simulink model "SS"  (R2017a)
settings: Solver=VariableStepAuto  StartTime=0.0  StopTime=50  RelTol=1e-3
values from neighbouring files (symbols this model uses):
  Ad = sysdd.A    [trock.m]
  Bd = sysdd.B(1:2)    [trock.m]
  C11 = [ C1(2,:); C1(4,:)]    [trock.m]
  Cd = sysdd.C    [trock.m]
  Dd = sysdd.D(:,1:2)    [trock.m]
  Ed = sysdd.B(3:4)    [trock.m]
  Kd = sysdd.D(:,3:4)    [trock.m]
  M_c = B_1 * A * B_1'    [trock.m]
  N_c = [ N(:,5) N(:,6)]    [trock.m]
  Ts = 0.566    [trock.m]
undefined symbols (not defined in the file or in its folder): Ac, Bc, Cc, Dc, Ec, Kc
libraries: powerlib_meascontrol x2
settings Model: Creator=CBalla  LastModifiedBy=nvink

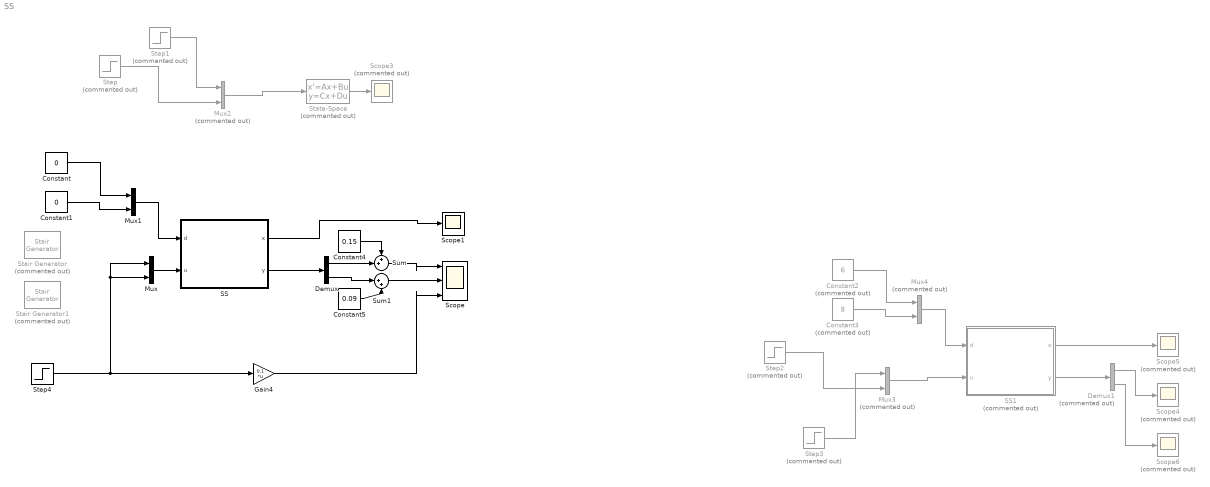
== system SS ==
  Constant : Constant  Value=0
  Constant1 : Constant  Value=0
  Constant2 : Constant  Commented=on  Value=6
  Constant3 : Constant  Commented=on  Value=8
  Constant4 : Constant  Value=0.15
  Constant5 : Constant  Value=0.09
  Demux : Demux  Outputs=2
  Demux1 : Demux  Commented=on  Outputs=2
  Gain4 : Gain  Gain=0.1  Multiplication=Matrix(K*u)
  Mux : Mux  Inputs=2
  Mux1 : Mux  Inputs=2
  Mux2 : Mux  Commented=on  Inputs=2
  Mux3 : Mux  Commented=on  Inputs=2
  Mux4 : Mux  Commented=on  Inputs=2
  SS : Subsystem
  SS1 : Subsystem  Commented=on
  Scope : Scope  NumInputPorts=3
  Scope1 : Scope
  Scope{3..6} (4 alike) : Scope  Commented=on
  Stair Generator : powerlib_meascontrol/Pulse & Signal Generators/Stair Generator  Commented=on  t=[0, 5, 10, 15, 20, 25, 30, 35, 40, 45]  e=[0, 1, 2, 3, 4 ,4 , 3, 2, 1,0]  Ts=0
      settings: SourceProductName=Simscape Power Systems
  Stair Generator1 : powerlib_meascontrol/Pulse & Signal Generators/Stair Generator  Commented=on  t=[0, 5, 10,15]  e=[0, 0.1, 0.2,0.4]  Ts=0
      settings: SourceProductName=Simscape Power Systems
  State-Space : StateSpace  Commented=on  A=-M_c  B=N_c  C=C11  D=[0, 0;0 ,0 ]  X0=0
  Step : Step  Commented=on  SampleTime=0
  Step1 : Step  Commented=on  Time=3  SampleTime=0
  Step2 : Step  Commented=on  SampleTime=0
  Step3 : Step  Commented=on  Time=15  SampleTime=0
  Step4 : Step  Time=5  After=0.4  SampleTime=0
  Sum : Sum  Inputs=++|
  Sum1 : Sum  Inputs=|++
  wires:
  SS/1(x) -> Scope1/1
  Mux/1 -> SS/2(u)
  Mux1/1 -> SS/1(d)
  Constant/1 -> Mux1/1
  Constant1/1 -> Mux1/2
  SS/2(y) -> Demux/1
  Mux2/1 -> State-Space/1
  State-Space/1 -> Scope3/1
  Step1/1 -> Mux2/1
  Step/1 -> Mux2/2
  SS1/1(x) -> Scope5/1
  Mux4/1 -> SS1/1(d)
  Constant2/1 -> Mux4/1
  Constant3/1 -> Mux4/2
  SS1/2(y) -> Demux1/1
  Demux1/1 -> Scope4/1
  Demux1/2 -> Scope6/1
  Mux3/1 -> SS1/2(u)
  Step3/1 -> Mux3/1
  Step2/1 -> Mux3/2
  Demux/1 -> Sum/2
  Demux/2 -> Sum1/1
  Constant4/1 -> Sum/1
  Constant5/1 -> Sum1/2
  Sum/1 -> Scope/1
  Sum1/1 -> Scope/2
  Step4/1 -> Gain4/1, Mux/1, Mux/2
  Gain4/1 -> Scope/3

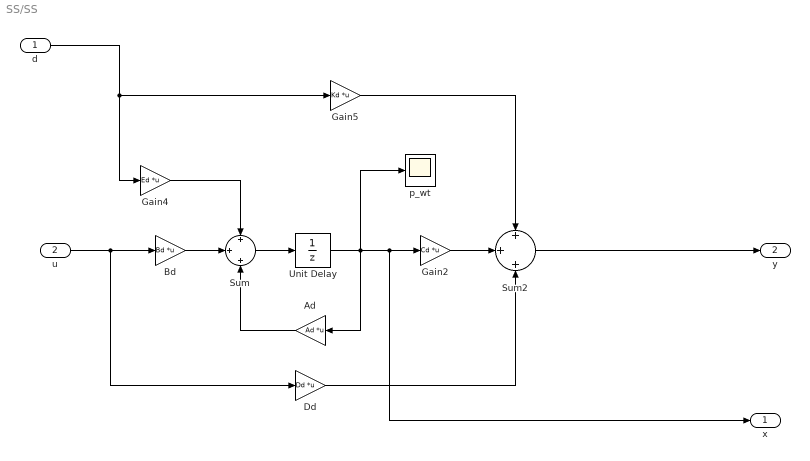
== system SS/SS ==
  d : Inport
  u : Inport  Port=2
  Ad : Gain  Gain=Ad  Multiplication=Matrix(K*u)
      mask Display:
      | %color('cyan')
      | color('magenta')
      | disp('{\bf\fontsize{14}Ad}', 'texmode','on');
      | %disp('Ad')
  Bd : Gain  Gain=Bd  Multiplication=Matrix(K*u)
      mask Display:
      | %color('cyan')
      | color('magenta')
      | disp('{\bf\fontsize{14}Bd}', 'texmode','on');
      | %disp('Bd')
  Dd : Gain  Gain=Dd  Multiplication=Matrix(K*u)
      mask Display:
      | %color('cyan')
      | color('magenta')
      | disp('{\bf\fontsize{14}Dd}', 'texmode','on');
      | %disp('Dd')
  Gain2 : Gain  Gain=Cd  Multiplication=Matrix(K*u)
      mask Display:
      | %color('cyan')
      | color('magenta')
      | disp('{\bf\fontsize{14}Cd}', 'texmode','on');
      | %disp('Cd')
  Gain4 : Gain  Gain=Ed  Multiplication=Matrix(K*u)
      mask Display:
      | %color('cyan')
      | color('magenta')
      | disp('{\bf\fontsize{14}Ed}', 'texmode','on');
      | %disp('Ed')
  Gain5 : Gain  Gain=Kd  Multiplication=Matrix(K*u)
      mask Display:
      | %color('cyan')
      | color('magenta')
      | disp('{\bf\fontsize{14}Kd}', 'texmode','on');
      | %disp('Kd')
  Sum : Sum  Inputs=+|+|+
  Sum2 : Sum  Inputs=+|+|+
  Unit Delay : UnitDelay  InitialCondition=0.005  SampleTime=Ts
  p_wt : Scope
  x : Outport
  y : Outport  Port=2
  wires:
  Sum2/1 -> y/1
  Sum/1 -> Unit Delay/1
  Bd/1 -> Sum/2
  Ad/1 -> Sum/3
  Unit Delay/1 -> p_wt/1, x/1, Gain2/1, Ad/1
  u/1 -> Dd/1, Bd/1
  d/1 -> Gain4/1, Gain5/1
  Gain2/1 -> Sum2/2
  Gain4/1 -> Sum/1
  Gain5/1 -> Sum2/1
  Dd/1 -> Sum2/3

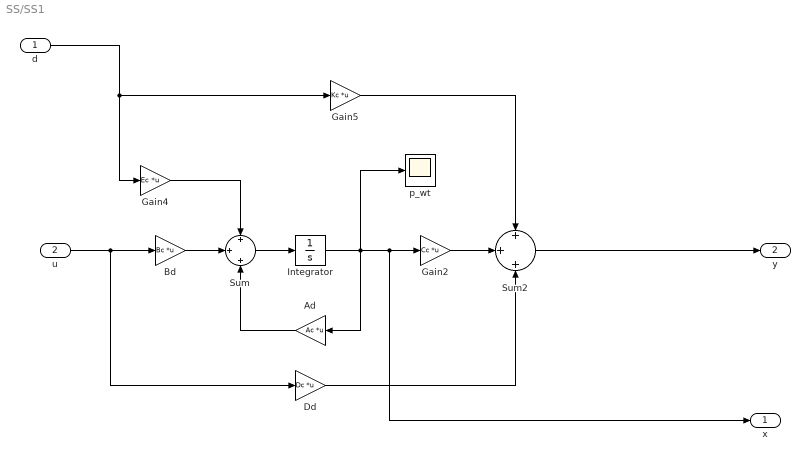
== system SS/SS1 ==
  d : Inport
  u : Inport  Port=2
  Ad : Gain  Gain=Ac  Multiplication=Matrix(K*u)
      mask Display:
      | %color('cyan')
      | color('magenta')
      | disp('{\bf\fontsize{14}Ad}', 'texmode','on');
      | %disp('Ad')
  Bd : Gain  Gain=Bc  Multiplication=Matrix(K*u)
      mask Display:
      | %color('cyan')
      | color('magenta')
      | disp('{\bf\fontsize{14}Bd}', 'texmode','on');
      | %disp('Bd')
  Dd : Gain  Gain=Dc  Multiplication=Matrix(K*u)
      mask Display:
      | %color('cyan')
      | color('magenta')
      | disp('{\bf\fontsize{14}Dd}', 'texmode','on');
      | %disp('Dd')
  Gain2 : Gain  Gain=Cc  Multiplication=Matrix(K*u)
      mask Display:
      | %color('cyan')
      | color('magenta')
      | disp('{\bf\fontsize{14}Cd}', 'texmode','on');
      | %disp('Cd')
  Gain4 : Gain  Gain=Ec  Multiplication=Matrix(K*u)
      mask Display:
      | %color('cyan')
      | color('magenta')
      | disp('{\bf\fontsize{14}Ed}', 'texmode','on');
      | %disp('Ed')
  Gain5 : Gain  Gain=Kc  Multiplication=Matrix(K*u)
      mask Display:
      | %color('cyan')
      | color('magenta')
      | disp('{\bf\fontsize{14}Kd}', 'texmode','on');
      | %disp('Kd')
  Integrator : Integrator
  Sum : Sum  Inputs=+|+|+
  Sum2 : Sum  Inputs=+|+|+
  p_wt : Scope
  x : Outport
  y : Outport  Port=2
  wires:
  Sum2/1 -> y/1
  Sum/1 -> Integrator/1
  Bd/1 -> Sum/2
  Ad/1 -> Sum/3
  Integrator/1 -> p_wt/1, x/1, Gain2/1, Ad/1
  u/1 -> Dd/1, Bd/1
  d/1 -> Gain4/1, Gain5/1
  Gain4/1 -> Sum/1
  Gain2/1 -> Sum2/2
  Dd/1 -> Sum2/3
  Gain5/1 -> Sum2/1
